simulink model "DiscretePolynomial"  (R2021a)
settings: Solver=FixedStepAuto  StartTime=0.0  StopTime=STime  FixedStep=1e-3  RelTol=1e-3
undefined symbols (not defined in the file): C, C_poly, cd_poly, denum_d, J, Kp, Mc, num_d, r0, R_poly, Ra, rd0, rd1, rd2, rd_poly, Ta, Tp, TPert, Tq
settings Model: Creator=akangmufti  LastModifiedBy=akangmufti

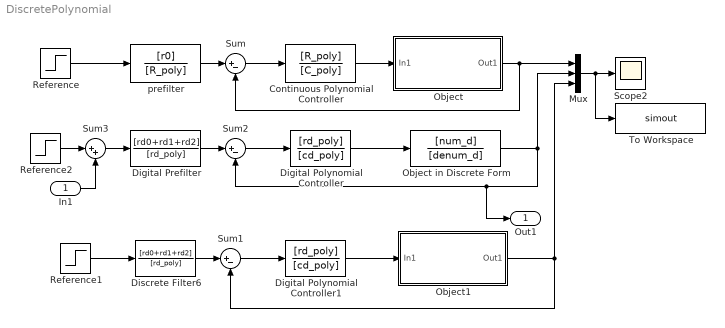
== system DiscretePolynomial ==
  In1 : Inport
  Continuous Polynomial Controller : TransferFcn  Numerator=[R_poly]  Denominator=[C_poly]
  Digital Polynomial Controller : DiscreteFilter  Numerator=[rd_poly]  Denominator=[cd_poly]  SampleTime=Tq
  Digital Polynomial Controller1 : DiscreteFilter  Numerator=[rd_poly]  Denominator=[cd_poly]  SampleTime=Tq
  Digital Prefilter : DiscreteFilter  Numerator=[rd0+rd1+rd2]  Denominator=[rd_poly]  SampleTime=Tq
  Discrete Filter6 : DiscreteFilter  Numerator=[rd0+rd1+rd2]  Denominator=[rd_poly]  SampleTime=Tq
  Mux : Mux  Inputs=3
  Object : Subsystem
  Object in Discrete Form : DiscreteTransferFcn  Numerator=[num_d]  Denominator=[denum_d]  SampleTime=Tq
  Object1 : Subsystem
  Reference : Step  Time=1e-3  SampleTime=0
  Reference1 : Step  Time=1e-3  SampleTime=0
  Reference2 : Step  Time=1e-3  SampleTime=0
  Scope2 : Scope
  Sum : Sum  Inputs=|+-
  Sum1 : Sum  Inputs=|+-
  Sum2 : Sum  Inputs=|+-
  Sum3 : Sum  Inputs=|++
  To Workspace : ToWorkspace  VariableName=simout  SampleTime=-1
  prefilter : TransferFcn  Numerator=[r0]  Denominator=[R_poly]
  Out1 : Outport
  wires:
  Object/1(Out1) -> Mux/1, Sum/2
  Sum/1 -> Continuous Polynomial Controller/1
  Continuous Polynomial Controller/1 -> Object/1(In1)
  Digital Polynomial Controller/1 -> Object in Discrete Form/1
  Sum2/1 -> Digital Polynomial Controller/1
  prefilter/1 -> Sum/1
  Reference/1 -> prefilter/1
  Sum1/1 -> Digital Polynomial Controller1/1
  Object1/1(Out1) -> Mux/3, Sum1/2
  Digital Prefilter/1 -> Sum2/1
  Discrete Filter6/1 -> Sum1/1
  Mux/1 -> Scope2/1, To Workspace/1
  Digital Polynomial Controller1/1 -> Object1/1(In1)
  Reference1/1 -> Discrete Filter6/1
  In1/1 -> Sum3/2
  Reference2/1 -> Sum3/1
  Sum3/1 -> Digital Prefilter/1
  Object in Discrete Form/1 -> Out1/1, Sum2/2, Mux/2

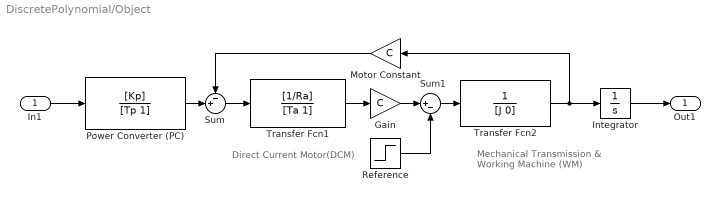
== system DiscretePolynomial/Object ==
  note: Direct Current Motor(DCM)
  note: Mechanical Transmission &
      | Working Machine (WM)
  In1 : Inport
  Gain : Gain  Gain=C
  Integrator : Integrator  ContinuousStateAttributes='AngularPosition'
  Motor Constant : Gain  Gain=C
  Power Converter (PC) : TransferFcn  Numerator=[Kp]  Denominator=[Tp 1]
  Reference : Step  Time=TPert  After=Mc  SampleTime=0
  Sum : Sum  Inputs=-+|
  Sum1 : Sum  Inputs=|+-
  Transfer Fcn1 : TransferFcn  Numerator=[1/Ra]  Denominator=[Ta 1]  ContinuousStateAttributes='Current'
  Transfer Fcn2 : TransferFcn  Denominator=[J 0]  ContinuousStateAttributes='Omega'
  Out1 : Outport
  wires:
  Transfer Fcn2/1 -> Integrator/1, Motor Constant/1
  Power Converter (PC)/1 -> Sum/2
  Gain/1 -> Sum1/1
  Sum1/1 -> Transfer Fcn2/1
  Sum/1 -> Transfer Fcn1/1
  Transfer Fcn1/1 -> Gain/1
  Motor Constant/1 -> Sum/1
  In1/1 -> Power Converter (PC)/1
  Reference/1 -> Sum1/2
  Integrator/1 -> Out1/1

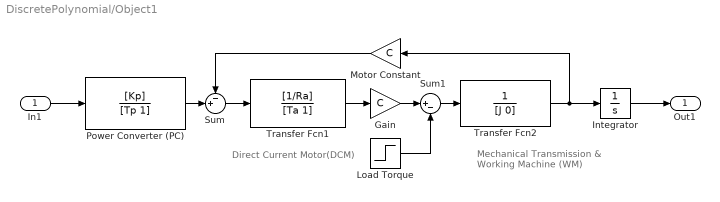
== system DiscretePolynomial/Object1 ==
  note: Direct Current Motor(DCM)
  note: Mechanical Transmission &
      | Working Machine (WM)
  In1 : Inport
  Gain : Gain  Gain=C
  Integrator : Integrator  ContinuousStateAttributes='AngularPosition'
  Load Torque : Step  Time=TPert  After=Mc  SampleTime=0
  Motor Constant : Gain  Gain=C
  Power Converter (PC) : TransferFcn  Numerator=[Kp]  Denominator=[Tp 1]
  Sum : Sum  Inputs=-+|
  Sum1 : Sum  Inputs=|+-
  Transfer Fcn1 : TransferFcn  Numerator=[1/Ra]  Denominator=[Ta 1]  ContinuousStateAttributes='Current'
  Transfer Fcn2 : TransferFcn  Denominator=[J 0]  ContinuousStateAttributes='Omega'
  Out1 : Outport
  wires:
  Transfer Fcn2/1 -> Integrator/1, Motor Constant/1
  Power Converter (PC)/1 -> Sum/2
  Gain/1 -> Sum1/1
  Sum1/1 -> Transfer Fcn2/1
  Sum/1 -> Transfer Fcn1/1
  Transfer Fcn1/1 -> Gain/1
  Motor Constant/1 -> Sum/1
  In1/1 -> Power Converter (PC)/1
  Load Torque/1 -> Sum1/2
  Integrator/1 -> Out1/1
